simulink model "FSAC2021"  (R2014a)
settings: Solver=FixedStepDiscrete  StartTime=0.0  StopTime=inf  FixedStep=0.0005  RelTol=1e-3
model workspace (MAT data in the model file):
  MCOS : class17 (value not decoded)
  MCOS : class17 (value not decoded)
  MCOS : class17 (value not decoded)
  MCOS : class17 (value not decoded)
  MCOS : class17 (value not decoded)
  MCOS : class17 (value not decoded)
  MCOS : class17 (value not decoded)
  MCOS : class17 (value not decoded)
  MCOS : class17 (value not decoded)
  MCOS : class17 (value not decoded)
  MCOS : class17 (value not decoded)
  MCOS : class17 (value not decoded)
  MCOS : class17 (value not decoded)
  MCOS : class17 (value not decoded)
  MCOS : class17 (value not decoded)
  MCOS : class17 (value not decoded)
  MCOS : class17 (value not decoded)
  MCOS : class17 (value not decoded)
  MCOS : class17 (value not decoded)
  BUZZER_START = 1
  MCOS : class17 (value not decoded)
  MCOS : class17 (value not decoded)
  MCOS : class17 (value not decoded)
  MCOS : class17 (value not decoded)
  MCOS : class17 (value not decoded)
  MCOS : class17 (value not decoded)
  MCOS : class17 (value not decoded)
  MCOS : class17 (value not decoded)
  MCOS : class17 (value not decoded)
  MCOS : class17 (value not decoded)
  MCOS : class17 (value not decoded)
  MCOS : class17 (value not decoded)
  MCOS : class17 (value not decoded)
  MCOS : class17 (value not decoded)
  MCOS : class17 (value not decoded)
  MCOS : class17 (value not decoded)
  MCOS : class17 (value not decoded)
  MCOS : class17 (value not decoded)
  MCOS : class17 (value not decoded)
  MCOS : class17 (value not decoded)
  MCOS : class17 (value not decoded)
  MCOS : class17 (value not decoded)
  MCOS : class17 (value not decoded)
  MCOS : class17 (value not decoded)
  MCOS : class17 (value not decoded)
  MCOS : class17 (value not decoded)
  MCOS : class17 (value not decoded)
  MCOS : class17 (value not decoded)
  MCOS : class17 (value not decoded)
  MCOS : class17 (value not decoded)
  MCOS : class17 (value not decoded)
  MCOS : class17 (value not decoded)
  MCOS : class17 (value not decoded)
  MCOS : class17 (value not decoded)
  MCOS : class17 (value not decoded)
  MCOS : class17 (value not decoded)
  MCOS : class17 (value not decoded)
  MCOS : class17 (value not decoded)
  Brake = 11
  MCOS : class17 (value not decoded)
  MCOS : class17 (value not decoded)
  MCOS : class17 (value not decoded)
  MCOS : class17 (value not decoded)
  MCOS : class17 (value not decoded)
  MCOS : class17 (value not decoded)
  MCOS : class17 (value not decoded)
  MCOS : class17 (value not decoded)
  Sensor_Acc_b = 101.85
  Sensor_Acc_k = -0.0185
  Str_Sen_Orig_Angle = -341
  MCOS : class17 (value not decoded)
  Tire_D = 0.47
  T = 0.05
libraries: simulink x396, ec55xxlib x126
(part 16 of 17)

== system FSAC2021/ROUTING/TO_DCAN/Subsystem/DIAG_VEH_INFO/EBS_Gas_SN_1_Sts ==
  EBS_Gas_SN_1_Sts : Inport
  Constant{1..3,5..8} (7 alike) : Constant  Value=0  OutDataTypeStr=uint8  SampleTime=-1
  EBS_Gas_SN_1_StsRon : Rounding  Operator=round
  EBS_Gas_SN_1_Sts_1sat : Saturate  UpperLimit=16  LowerLimit=0
  EBS_Gas_SN_1_Sts_Convert : DataTypeConversion  OutDataTypeStr=uint8
  EBS_Gas_SN_1_Sts_Convert1 : DataTypeConversion  OutDataTypeStr=uint32
  EBS_Gas_SN_1_Sts_D : Product  Inputs=*/
  EBS_Gas_SN_1_Sts_F : Constant  OutDataTypeStr=single
  EBS_Gas_SN_1_Sts_L : simulink/Logic and Bit Operations/Bitwise Operator  logicop=AND  UseBitMask=on  BitMask=16  BitMaskRealWorld=Stored Integer
  EBS_Gas_SN_1_Sts_O : Constant  Value=0  OutDataTypeStr=single
  EBS_Gas_SN_1_Sts_S : ArithShift  BitShiftNumber=-4
  EBS_Gas_SN_1_Sts_sat : Saturate  UpperLimit=1  LowerLimit=0
  EBS_Gas_SN_1_Sts_st : Sum  Inputs=+-
  output1 : Outport
  output2 : Outport  Port=2
  output3 : Outport  Port=3
  output4 : Outport  Port=4
  output5 : Outport  Port=5
  output6 : Outport  Port=6
  output7 : Outport  Port=7
  output8 : Outport  Port=8
  wires:
  EBS_Gas_SN_1_Sts/1 -> EBS_Gas_SN_1_Sts_sat/1
  EBS_Gas_SN_1_Sts_sat/1 -> EBS_Gas_SN_1_Sts_st/1
  EBS_Gas_SN_1_Sts_O/1 -> EBS_Gas_SN_1_Sts_st/2
  EBS_Gas_SN_1_Sts_st/1 -> EBS_Gas_SN_1_Sts_D/1
  EBS_Gas_SN_1_Sts_F/1 -> EBS_Gas_SN_1_Sts_D/2
  EBS_Gas_SN_1_Sts_D/1 -> EBS_Gas_SN_1_StsRon/1
  EBS_Gas_SN_1_StsRon/1 -> EBS_Gas_SN_1_Sts_S/1
  EBS_Gas_SN_1_Sts_S/1 -> EBS_Gas_SN_1_Sts_1sat/1
  EBS_Gas_SN_1_Sts_1sat/1 -> EBS_Gas_SN_1_Sts_Convert1/1
  EBS_Gas_SN_1_Sts_Convert1/1 -> EBS_Gas_SN_1_Sts_L/1
  EBS_Gas_SN_1_Sts_L/1 -> EBS_Gas_SN_1_Sts_Convert/1
  EBS_Gas_SN_1_Sts_Convert/1 -> output4/1
  Constant1/1 -> output1/1
  Constant2/1 -> output2/1
  Constant3/1 -> output3/1
  Constant5/1 -> output5/1
  Constant6/1 -> output6/1
  Constant7/1 -> output7/1
  Constant8/1 -> output8/1

== system FSAC2021/ROUTING/TO_DCAN/Subsystem/DIAG_VEH_INFO/EBS_Gas_SN_2_Sts ==
  EBS_Gas_SN_2_Sts : Inport
  Constant{1..3,5..8} (7 alike) : Constant  Value=0  OutDataTypeStr=uint8  SampleTime=-1
  EBS_Gas_SN_2_StsRon : Rounding  Operator=round
  EBS_Gas_SN_2_Sts_1sat : Saturate  UpperLimit=8  LowerLimit=0
  EBS_Gas_SN_2_Sts_Convert : DataTypeConversion  OutDataTypeStr=uint8
  EBS_Gas_SN_2_Sts_Convert1 : DataTypeConversion  OutDataTypeStr=uint32
  EBS_Gas_SN_2_Sts_D : Product  Inputs=*/
  EBS_Gas_SN_2_Sts_F : Constant  OutDataTypeStr=single
  EBS_Gas_SN_2_Sts_L : simulink/Logic and Bit Operations/Bitwise Operator  logicop=AND  UseBitMask=on  BitMask=8  BitMaskRealWorld=Stored Integer
  EBS_Gas_SN_2_Sts_O : Constant  Value=0  OutDataTypeStr=single
  EBS_Gas_SN_2_Sts_S : ArithShift  BitShiftNumber=-3
  EBS_Gas_SN_2_Sts_sat : Saturate  UpperLimit=1  LowerLimit=0
  EBS_Gas_SN_2_Sts_st : Sum  Inputs=+-
  output1 : Outport
  output2 : Outport  Port=2
  output3 : Outport  Port=3
  output4 : Outport  Port=4
  output5 : Outport  Port=5
  output6 : Outport  Port=6
  output7 : Outport  Port=7
  output8 : Outport  Port=8
  wires:
  EBS_Gas_SN_2_Sts/1 -> EBS_Gas_SN_2_Sts_sat/1
  EBS_Gas_SN_2_Sts_sat/1 -> EBS_Gas_SN_2_Sts_st/1
  EBS_Gas_SN_2_Sts_O/1 -> EBS_Gas_SN_2_Sts_st/2
  EBS_Gas_SN_2_Sts_st/1 -> EBS_Gas_SN_2_Sts_D/1
  EBS_Gas_SN_2_Sts_F/1 -> EBS_Gas_SN_2_Sts_D/2
  EBS_Gas_SN_2_Sts_D/1 -> EBS_Gas_SN_2_StsRon/1
  EBS_Gas_SN_2_StsRon/1 -> EBS_Gas_SN_2_Sts_S/1
  EBS_Gas_SN_2_Sts_S/1 -> EBS_Gas_SN_2_Sts_1sat/1
  EBS_Gas_SN_2_Sts_1sat/1 -> EBS_Gas_SN_2_Sts_Convert1/1
  EBS_Gas_SN_2_Sts_Convert1/1 -> EBS_Gas_SN_2_Sts_L/1
  EBS_Gas_SN_2_Sts_L/1 -> EBS_Gas_SN_2_Sts_Convert/1
  EBS_Gas_SN_2_Sts_Convert/1 -> output4/1
  Constant1/1 -> output1/1
  Constant2/1 -> output2/1
  Constant3/1 -> output3/1
  Constant5/1 -> output5/1
  Constant6/1 -> output6/1
  Constant7/1 -> output7/1
  Constant8/1 -> output8/1

== system FSAC2021/ROUTING/TO_DCAN/Subsystem/DIAG_VEH_INFO/EBS_Rls_Switch ==
  EBS_Rls_Switch : Inport
  Constant{1,3..8} (7 alike) : Constant  Value=0  OutDataTypeStr=uint8  SampleTime=-1
  EBS_Rls_SwitchRon : Rounding  Operator=round
  EBS_Rls_Switch_1sat : Saturate  UpperLimit=8  LowerLimit=0
  EBS_Rls_Switch_Convert : DataTypeConversion  OutDataTypeStr=uint8
  EBS_Rls_Switch_Convert1 : DataTypeConversion  OutDataTypeStr=uint32
  EBS_Rls_Switch_D : Product  Inputs=*/
  EBS_Rls_Switch_F : Constant  OutDataTypeStr=single
  EBS_Rls_Switch_L : simulink/Logic and Bit Operations/Bitwise Operator  logicop=AND  UseBitMask=on  BitMask=8  BitMaskRealWorld=Stored Integer
  EBS_Rls_Switch_O : Constant  Value=0  OutDataTypeStr=single
  EBS_Rls_Switch_S : ArithShift  BitShiftNumber=-3
  EBS_Rls_Switch_sat : Saturate  UpperLimit=1  LowerLimit=0
  EBS_Rls_Switch_st : Sum  Inputs=+-
  output1 : Outport
  output2 : Outport  Port=2
  output3 : Outport  Port=3
  output4 : Outport  Port=4
  output5 : Outport  Port=5
  output6 : Outport  Port=6
  output7 : Outport  Port=7
  output8 : Outport  Port=8
  wires:
  EBS_Rls_Switch/1 -> EBS_Rls_Switch_sat/1
  EBS_Rls_Switch_sat/1 -> EBS_Rls_Switch_st/1
  EBS_Rls_Switch_O/1 -> EBS_Rls_Switch_st/2
  EBS_Rls_Switch_st/1 -> EBS_Rls_Switch_D/1
  EBS_Rls_Switch_F/1 -> EBS_Rls_Switch_D/2
  EBS_Rls_Switch_D/1 -> EBS_Rls_SwitchRon/1
  EBS_Rls_SwitchRon/1 -> EBS_Rls_Switch_S/1
  EBS_Rls_Switch_S/1 -> EBS_Rls_Switch_1sat/1
  EBS_Rls_Switch_1sat/1 -> EBS_Rls_Switch_Convert1/1
  EBS_Rls_Switch_Convert1/1 -> EBS_Rls_Switch_L/1
  EBS_Rls_Switch_L/1 -> EBS_Rls_Switch_Convert/1
  EBS_Rls_Switch_Convert/1 -> output2/1
  Constant1/1 -> output1/1
  Constant3/1 -> output3/1
  Constant4/1 -> output4/1
  Constant5/1 -> output5/1
  Constant6/1 -> output6/1
  Constant7/1 -> output7/1
  Constant8/1 -> output8/1

== system FSAC2021/ROUTING/TO_DCAN/Subsystem/DIAG_VEH_INFO/EBS_Status ==
  EBS_Status : Inport
  Constant{2..8} (7 alike) : Constant  Value=0  OutDataTypeStr=uint8  SampleTime=-1
  EBS_StatusRon : Rounding  Operator=round
  EBS_Status_1sat : Saturate  UpperLimit=192  LowerLimit=0
  EBS_Status_Convert : DataTypeConversion  OutDataTypeStr=uint8
  EBS_Status_Convert1 : DataTypeConversion  OutDataTypeStr=uint32
  EBS_Status_D : Product  Inputs=*/
  EBS_Status_F : Constant  OutDataTypeStr=single
  EBS_Status_L : simulink/Logic and Bit Operations/Bitwise Operator  logicop=AND  UseBitMask=on  BitMask=192  BitMaskRealWorld=Stored Integer
  EBS_Status_O : Constant  Value=0  OutDataTypeStr=single
  EBS_Status_S : ArithShift  BitShiftNumber=-6
  EBS_Status_sat : Saturate  UpperLimit=3  LowerLimit=0
  EBS_Status_st : Sum  Inputs=+-
  output1 : Outport
  output2 : Outport  Port=2
  output3 : Outport  Port=3
  output4 : Outport  Port=4
  output5 : Outport  Port=5
  output6 : Outport  Port=6
  output7 : Outport  Port=7
  output8 : Outport  Port=8
  wires:
  EBS_Status/1 -> EBS_Status_sat/1
  EBS_Status_sat/1 -> EBS_Status_st/1
  EBS_Status_O/1 -> EBS_Status_st/2
  EBS_Status_st/1 -> EBS_Status_D/1
  EBS_Status_F/1 -> EBS_Status_D/2
  EBS_Status_D/1 -> EBS_StatusRon/1
  EBS_StatusRon/1 -> EBS_Status_S/1
  EBS_Status_S/1 -> EBS_Status_1sat/1
  EBS_Status_1sat/1 -> EBS_Status_Convert1/1
  EBS_Status_Convert1/1 -> EBS_Status_L/1
  EBS_Status_L/1 -> EBS_Status_Convert/1
  EBS_Status_Convert/1 -> output1/1
  Constant2/1 -> output2/1
  Constant3/1 -> output3/1
  Constant4/1 -> output4/1
  Constant5/1 -> output5/1
  Constant6/1 -> output6/1
  Constant7/1 -> output7/1
  Constant8/1 -> output8/1

== system FSAC2021/ROUTING/TO_DCAN/Subsystem/DIAG_VEH_INFO/HV_Switch ==
  HV_Switch : Inport
  Constant{1,3..8} (7 alike) : Constant  Value=0  OutDataTypeStr=uint8  SampleTime=-1
  HV_SwitchRon : Rounding  Operator=round
  HV_Switch_1sat : Saturate  UpperLimit=16  LowerLimit=0
  HV_Switch_Convert : DataTypeConversion  OutDataTypeStr=uint8
  HV_Switch_Convert1 : DataTypeConversion  OutDataTypeStr=uint32
  HV_Switch_D : Product  Inputs=*/
  HV_Switch_F : Constant  OutDataTypeStr=single
  HV_Switch_L : simulink/Logic and Bit Operations/Bitwise Operator  logicop=AND  UseBitMask=on  BitMask=16  BitMaskRealWorld=Stored Integer
  HV_Switch_O : Constant  Value=0  OutDataTypeStr=single
  HV_Switch_S : ArithShift  BitShiftNumber=-4
  HV_Switch_sat : Saturate  UpperLimit=1  LowerLimit=0
  HV_Switch_st : Sum  Inputs=+-
  output1 : Outport
  output2 : Outport  Port=2
  output3 : Outport  Port=3
  output4 : Outport  Port=4
  output5 : Outport  Port=5
  output6 : Outport  Port=6
  output7 : Outport  Port=7
  output8 : Outport  Port=8
  wires:
  HV_Switch/1 -> HV_Switch_sat/1
  HV_Switch_sat/1 -> HV_Switch_st/1
  HV_Switch_O/1 -> HV_Switch_st/2
  HV_Switch_st/1 -> HV_Switch_D/1
  HV_Switch_F/1 -> HV_Switch_D/2
  HV_Switch_D/1 -> HV_SwitchRon/1
  HV_SwitchRon/1 -> HV_Switch_S/1
  HV_Switch_S/1 -> HV_Switch_1sat/1
  HV_Switch_1sat/1 -> HV_Switch_Convert1/1
  HV_Switch_Convert1/1 -> HV_Switch_L/1
  HV_Switch_L/1 -> HV_Switch_Convert/1
  HV_Switch_Convert/1 -> output2/1
  Constant1/1 -> output1/1
  Constant3/1 -> output3/1
  Constant4/1 -> output4/1
  Constant5/1 -> output5/1
  Constant6/1 -> output6/1
  Constant7/1 -> output7/1
  Constant8/1 -> output8/1

== system FSAC2021/ROUTING/TO_DCAN/Subsystem/DIAG_VEH_INFO/High_voltage_on ==
  High_voltage_on : Inport
  Constant{1,3..8} (7 alike) : Constant  Value=0  OutDataTypeStr=uint8  SampleTime=-1
  High_voltage_onRon : Rounding  Operator=round
  High_voltage_on_1sat : Saturate  UpperLimit=2  LowerLimit=0
  High_voltage_on_Convert : DataTypeConversion  OutDataTypeStr=uint8
  High_voltage_on_Convert1 : DataTypeConversion  OutDataTypeStr=uint32
  High_voltage_on_D : Product  Inputs=*/
  High_voltage_on_F : Constant  OutDataTypeStr=single
  High_voltage_on_L : simulink/Logic and Bit Operations/Bitwise Operator  logicop=AND  UseBitMask=on  BitMask=2  BitMaskRealWorld=Stored Integer
  High_voltage_on_O : Constant  Value=0  OutDataTypeStr=single
  High_voltage_on_S : ArithShift  BitShiftNumber=-1
  High_voltage_on_sat : Saturate  UpperLimit=1  LowerLimit=0
  High_voltage_on_st : Sum  Inputs=+-
  output1 : Outport
  output2 : Outport  Port=2
  output3 : Outport  Port=3
  output4 : Outport  Port=4
  output5 : Outport  Port=5
  output6 : Outport  Port=6
  output7 : Outport  Port=7
  output8 : Outport  Port=8
  wires:
  High_voltage_on/1 -> High_voltage_on_sat/1
  High_voltage_on_sat/1 -> High_voltage_on_st/1
  High_voltage_on_O/1 -> High_voltage_on_st/2
  High_voltage_on_st/1 -> High_voltage_on_D/1
  High_voltage_on_F/1 -> High_voltage_on_D/2
  High_voltage_on_D/1 -> High_voltage_onRon/1
  High_voltage_onRon/1 -> High_voltage_on_S/1
  High_voltage_on_S/1 -> High_voltage_on_1sat/1
  High_voltage_on_1sat/1 -> High_voltage_on_Convert1/1
  High_voltage_on_Convert1/1 -> High_voltage_on_L/1
  High_voltage_on_L/1 -> High_voltage_on_Convert/1
  High_voltage_on_Convert/1 -> output2/1
  Constant1/1 -> output1/1
  Constant3/1 -> output3/1
  Constant4/1 -> output4/1
  Constant5/1 -> output5/1
  Constant6/1 -> output6/1
  Constant7/1 -> output7/1
  Constant8/1 -> output8/1

== system FSAC2021/ROUTING/TO_DCAN/Subsystem/DIAG_VEH_INFO/Hydra_Prs_SN_Sts ==
  Hydra_Prs_SN_Sts : Inport
  Constant{2..8} (7 alike) : Constant  Value=0  OutDataTypeStr=uint8  SampleTime=-1
  Hydra_Prs_SN_StsRon : Rounding  Operator=round
  Hydra_Prs_SN_Sts_1sat : Saturate  UpperLimit=1  LowerLimit=0
  Hydra_Prs_SN_Sts_Convert : DataTypeConversion  OutDataTypeStr=uint8
  Hydra_Prs_SN_Sts_Convert1 : DataTypeConversion  OutDataTypeStr=uint32
  Hydra_Prs_SN_Sts_D : Product  Inputs=*/
  Hydra_Prs_SN_Sts_F : Constant  OutDataTypeStr=single
  Hydra_Prs_SN_Sts_L : simulink/Logic and Bit Operations/Bitwise Operator  logicop=AND  UseBitMask=on  BitMask=1  BitMaskRealWorld=Stored Integer
  Hydra_Prs_SN_Sts_O : Constant  Value=0  OutDataTypeStr=single
  Hydra_Prs_SN_Sts_S : ArithShift
  Hydra_Prs_SN_Sts_sat : Saturate  UpperLimit=1  LowerLimit=0
  Hydra_Prs_SN_Sts_st : Sum  Inputs=+-
  output1 : Outport
  output2 : Outport  Port=2
  output3 : Outport  Port=3
  output4 : Outport  Port=4
  output5 : Outport  Port=5
  output6 : Outport  Port=6
  output7 : Outport  Port=7
  output8 : Outport  Port=8
  wires:
  Hydra_Prs_SN_Sts/1 -> Hydra_Prs_SN_Sts_sat/1
  Hydra_Prs_SN_Sts_sat/1 -> Hydra_Prs_SN_Sts_st/1
  Hydra_Prs_SN_Sts_O/1 -> Hydra_Prs_SN_Sts_st/2
  Hydra_Prs_SN_Sts_st/1 -> Hydra_Prs_SN_Sts_D/1
  Hydra_Prs_SN_Sts_F/1 -> Hydra_Prs_SN_Sts_D/2
  Hydra_Prs_SN_Sts_D/1 -> Hydra_Prs_SN_StsRon/1
  Hydra_Prs_SN_StsRon/1 -> Hydra_Prs_SN_Sts_S/1
  Hydra_Prs_SN_Sts_S/1 -> Hydra_Prs_SN_Sts_1sat/1
  Hydra_Prs_SN_Sts_1sat/1 -> Hydra_Prs_SN_Sts_Convert1/1
  Hydra_Prs_SN_Sts_Convert1/1 -> Hydra_Prs_SN_Sts_L/1
  Hydra_Prs_SN_Sts_L/1 -> Hydra_Prs_SN_Sts_Convert/1
  Hydra_Prs_SN_Sts_Convert/1 -> output1/1
  Constant2/1 -> output2/1
  Constant3/1 -> output3/1
  Constant4/1 -> output4/1
  Constant5/1 -> output5/1
  Constant6/1 -> output6/1
  Constant7/1 -> output7/1
  Constant8/1 -> output8/1

== system FSAC2021/ROUTING/TO_DCAN/Subsystem/DIAG_VEH_INFO/LV_Switch ==
  LV_Switch : Inport
  Constant{1,3..8} (7 alike) : Constant  Value=0  OutDataTypeStr=uint8  SampleTime=-1
  LV_SwitchRon : Rounding  Operator=round
  LV_Switch_1sat : Saturate  UpperLimit=32  LowerLimit=0
  LV_Switch_Convert : DataTypeConversion  OutDataTypeStr=uint8
  LV_Switch_Convert1 : DataTypeConversion  OutDataTypeStr=uint32
  LV_Switch_D : Product  Inputs=*/
  LV_Switch_F : Constant  OutDataTypeStr=single
  LV_Switch_L : simulink/Logic and Bit Operations/Bitwise Operator  logicop=AND  UseBitMask=on  BitMask=32  BitMaskRealWorld=Stored Integer
  LV_Switch_O : Constant  Value=0  OutDataTypeStr=single
  LV_Switch_S : ArithShift  BitShiftNumber=-5
  LV_Switch_sat : Saturate  UpperLimit=1  LowerLimit=0
  LV_Switch_st : Sum  Inputs=+-
  output1 : Outport
  output2 : Outport  Port=2
  output3 : Outport  Port=3
  output4 : Outport  Port=4
  output5 : Outport  Port=5
  output6 : Outport  Port=6
  output7 : Outport  Port=7
  output8 : Outport  Port=8
  wires:
  LV_Switch/1 -> LV_Switch_sat/1
  LV_Switch_sat/1 -> LV_Switch_st/1
  LV_Switch_O/1 -> LV_Switch_st/2
  LV_Switch_st/1 -> LV_Switch_D/1
  LV_Switch_F/1 -> LV_Switch_D/2
  LV_Switch_D/1 -> LV_SwitchRon/1
  LV_SwitchRon/1 -> LV_Switch_S/1
  LV_Switch_S/1 -> LV_Switch_1sat/1
  LV_Switch_1sat/1 -> LV_Switch_Convert1/1
  LV_Switch_Convert1/1 -> LV_Switch_L/1
  LV_Switch_L/1 -> LV_Switch_Convert/1
  LV_Switch_Convert/1 -> output2/1
  Constant1/1 -> output1/1
  Constant3/1 -> output3/1
  Constant4/1 -> output4/1
  Constant5/1 -> output5/1
  Constant6/1 -> output6/1
  Constant7/1 -> output7/1
  Constant8/1 -> output8/1

== system FSAC2021/ROUTING/TO_DCAN/Subsystem/DIAG_VEH_INFO/On_In_Swtich ==
  On_In_Swtich : Inport
  Constant{1,3..8} (7 alike) : Constant  Value=0  OutDataTypeStr=uint8  SampleTime=-1
  On_In_SwtichRon : Rounding  Operator=round
  On_In_Swtich_1sat : Saturate  UpperLimit=64  LowerLimit=0
  On_In_Swtich_Convert : DataTypeConversion  OutDataTypeStr=uint8
  On_In_Swtich_Convert1 : DataTypeConversion  OutDataTypeStr=uint32
  On_In_Swtich_D : Product  Inputs=*/
  On_In_Swtich_F : Constant  OutDataTypeStr=single
  On_In_Swtich_L : simulink/Logic and Bit Operations/Bitwise Operator  logicop=AND  UseBitMask=on  BitMask=64  BitMaskRealWorld=Stored Integer
  On_In_Swtich_O : Constant  Value=0  OutDataTypeStr=single
  On_In_Swtich_S : ArithShift  BitShiftNumber=-6
  On_In_Swtich_sat : Saturate  UpperLimit=1  LowerLimit=0
  On_In_Swtich_st : Sum  Inputs=+-
  output1 : Outport
  output2 : Outport  Port=2
  output3 : Outport  Port=3
  output4 : Outport  Port=4
  output5 : Outport  Port=5
  output6 : Outport  Port=6
  output7 : Outport  Port=7
  output8 : Outport  Port=8
  wires:
  On_In_Swtich/1 -> On_In_Swtich_sat/1
  On_In_Swtich_sat/1 -> On_In_Swtich_st/1
  On_In_Swtich_O/1 -> On_In_Swtich_st/2
  On_In_Swtich_st/1 -> On_In_Swtich_D/1
  On_In_Swtich_F/1 -> On_In_Swtich_D/2
  On_In_Swtich_D/1 -> On_In_SwtichRon/1
  On_In_SwtichRon/1 -> On_In_Swtich_S/1
  On_In_Swtich_S/1 -> On_In_Swtich_1sat/1
  On_In_Swtich_1sat/1 -> On_In_Swtich_Convert1/1
  On_In_Swtich_Convert1/1 -> On_In_Swtich_L/1
  On_In_Swtich_L/1 -> On_In_Swtich_Convert/1
  On_In_Swtich_Convert/1 -> output2/1
  Constant1/1 -> output1/1
  Constant3/1 -> output3/1
  Constant4/1 -> output4/1
  Constant5/1 -> output5/1
  Constant6/1 -> output6/1
  Constant7/1 -> output7/1
  Constant8/1 -> output8/1

== system FSAC2021/ROUTING/TO_DCAN/Subsystem/DIAG_VEH_INFO/On_Out_Switch ==
  On_Out_Switch : Inport
  Constant{1,3..8} (7 alike) : Constant  Value=0  OutDataTypeStr=uint8  SampleTime=-1
  On_Out_SwitchRon : Rounding  Operator=round
  On_Out_Switch_1sat : Saturate  UpperLimit=128  LowerLimit=0
  On_Out_Switch_Convert : DataTypeConversion  OutDataTypeStr=uint8
  On_Out_Switch_Convert1 : DataTypeConversion  OutDataTypeStr=uint32
  On_Out_Switch_D : Product  Inputs=*/
  On_Out_Switch_F : Constant  OutDataTypeStr=single
  On_Out_Switch_L : simulink/Logic and Bit Operations/Bitwise Operator  logicop=AND  UseBitMask=on  BitMask=128  BitMaskRealWorld=Stored Integer
  On_Out_Switch_O : Constant  Value=0  OutDataTypeStr=single
  On_Out_Switch_S : ArithShift  BitShiftNumber=-7
  On_Out_Switch_sat : Saturate  UpperLimit=1  LowerLimit=0
  On_Out_Switch_st : Sum  Inputs=+-
  output1 : Outport
  output2 : Outport  Port=2
  output3 : Outport  Port=3
  output4 : Outport  Port=4
  output5 : Outport  Port=5
  output6 : Outport  Port=6
  output7 : Outport  Port=7
  output8 : Outport  Port=8
  wires:
  On_Out_Switch/1 -> On_Out_Switch_sat/1
  On_Out_Switch_sat/1 -> On_Out_Switch_st/1
  On_Out_Switch_O/1 -> On_Out_Switch_st/2
  On_Out_Switch_st/1 -> On_Out_Switch_D/1
  On_Out_Switch_F/1 -> On_Out_Switch_D/2
  On_Out_Switch_D/1 -> On_Out_SwitchRon/1
  On_Out_SwitchRon/1 -> On_Out_Switch_S/1
  On_Out_Switch_S/1 -> On_Out_Switch_1sat/1
  On_Out_Switch_1sat/1 -> On_Out_Switch_Convert1/1
  On_Out_Switch_Convert1/1 -> On_Out_Switch_L/1
  On_Out_Switch_L/1 -> On_Out_Switch_Convert/1
  On_Out_Switch_Convert/1 -> output2/1
  Constant1/1 -> output1/1
  Constant3/1 -> output3/1
  Constant4/1 -> output4/1
  Constant5/1 -> output5/1
  Constant6/1 -> output6/1
  Constant7/1 -> output7/1
  Constant8/1 -> output8/1

== system FSAC2021/ROUTING/TO_DCAN/Subsystem/DIAG_VEH_INFO/Point_BCU ==
  Point_BCU : Inport
  Constant{1..2,4..8} (7 alike) : Constant  Value=0  OutDataTypeStr=uint8  SampleTime=-1
  Point_BCURon : Rounding  Operator=round
  Point_BCU_1sat : Saturate  UpperLimit=32  LowerLimit=0
  Point_BCU_Convert : DataTypeConversion  OutDataTypeStr=uint8
  Point_BCU_Convert1 : DataTypeConversion  OutDataTypeStr=uint32
  Point_BCU_D : Product  Inputs=*/
  Point_BCU_F : Constant  OutDataTypeStr=single
  Point_BCU_L : simulink/Logic and Bit Operations/Bitwise Operator  logicop=AND  UseBitMask=on  BitMask=32  BitMaskRealWorld=Stored Integer
  Point_BCU_O : Constant  Value=0  OutDataTypeStr=single
  Point_BCU_S : ArithShift  BitShiftNumber=-5
  Point_BCU_sat : Saturate  UpperLimit=1  LowerLimit=0
  Point_BCU_st : Sum  Inputs=+-
  output1 : Outport
  output2 : Outport  Port=2
  output3 : Outport  Port=3
  output4 : Outport  Port=4
  output5 : Outport  Port=5
  output6 : Outport  Port=6
  output7 : Outport  Port=7
  output8 : Outport  Port=8
  wires:
  Point_BCU/1 -> Point_BCU_sat/1
  Point_BCU_sat/1 -> Point_BCU_st/1
  Point_BCU_O/1 -> Point_BCU_st/2
  Point_BCU_st/1 -> Point_BCU_D/1
  Point_BCU_F/1 -> Point_BCU_D/2
  Point_BCU_D/1 -> Point_BCURon/1
  Point_BCURon/1 -> Point_BCU_S/1
  Point_BCU_S/1 -> Point_BCU_1sat/1
  Point_BCU_1sat/1 -> Point_BCU_Convert1/1
  Point_BCU_Convert1/1 -> Point_BCU_L/1
  Point_BCU_L/1 -> Point_BCU_Convert/1
  Point_BCU_Convert/1 -> output3/1
  Constant1/1 -> output1/1
  Constant2/1 -> output2/1
  Constant4/1 -> output4/1
  Constant5/1 -> output5/1
  Constant6/1 -> output6/1
  Constant7/1 -> output7/1
  Constant8/1 -> output8/1

== system FSAC2021/ROUTING/TO_DCAN/Subsystem/DIAG_VEH_INFO/Point_BMS ==
  Point_BMS : Inport
  Constant{1..2,4..8} (7 alike) : Constant  Value=0  OutDataTypeStr=uint8  SampleTime=-1
  Point_BMSRon : Rounding  Operator=round
  Point_BMS_1sat : Saturate  UpperLimit=16  LowerLimit=0
  Point_BMS_Convert : DataTypeConversion  OutDataTypeStr=uint8
  Point_BMS_Convert1 : DataTypeConversion  OutDataTypeStr=uint32
  Point_BMS_D : Product  Inputs=*/
  Point_BMS_F : Constant  OutDataTypeStr=single
  Point_BMS_L : simulink/Logic and Bit Operations/Bitwise Operator  logicop=AND  UseBitMask=on  BitMask=16  BitMaskRealWorld=Stored Integer
  Point_BMS_O : Constant  Value=0  OutDataTypeStr=single
  Point_BMS_S : ArithShift  BitShiftNumber=-4
  Point_BMS_sat : Saturate  UpperLimit=1  LowerLimit=0
  Point_BMS_st : Sum  Inputs=+-
  output1 : Outport
  output2 : Outport  Port=2
  output3 : Outport  Port=3
  output4 : Outport  Port=4
  output5 : Outport  Port=5
  output6 : Outport  Port=6
  output7 : Outport  Port=7
  output8 : Outport  Port=8
  wires:
  Point_BMS/1 -> Point_BMS_sat/1
  Point_BMS_sat/1 -> Point_BMS_st/1
  Point_BMS_O/1 -> Point_BMS_st/2
  Point_BMS_st/1 -> Point_BMS_D/1
  Point_BMS_F/1 -> Point_BMS_D/2
  Point_BMS_D/1 -> Point_BMSRon/1
  Point_BMSRon/1 -> Point_BMS_S/1
  Point_BMS_S/1 -> Point_BMS_1sat/1
  Point_BMS_1sat/1 -> Point_BMS_Convert1/1
  Point_BMS_Convert1/1 -> Point_BMS_L/1
  Point_BMS_L/1 -> Point_BMS_Convert/1
  Point_BMS_Convert/1 -> output3/1
  Constant1/1 -> output1/1
  Constant2/1 -> output2/1
  Constant4/1 -> output4/1
  Constant5/1 -> output5/1
  Constant6/1 -> output6/1
  Constant7/1 -> output7/1
  Constant8/1 -> output8/1

== system FSAC2021/ROUTING/TO_DCAN/Subsystem/DIAG_VEH_INFO/Point_Drive_Motor ==
  Point_Drive_Motor : Inport
  Constant{1..2,4..8} (7 alike) : Constant  Value=0  OutDataTypeStr=uint8  SampleTime=-1
  Point_Drive_MotorRon : Rounding  Operator=round
  Point_Drive_Motor_1sat : Saturate  UpperLimit=8  LowerLimit=0
  Point_Drive_Motor_Convert : DataTypeConversion  OutDataTypeStr=uint8
  Point_Drive_Motor_Convert1 : DataTypeConversion  OutDataTypeStr=uint32
  Point_Drive_Motor_D : Product  Inputs=*/
  Point_Drive_Motor_F : Constant  OutDataTypeStr=single
  Point_Drive_Motor_L : simulink/Logic and Bit Operations/Bitwise Operator  logicop=AND  UseBitMask=on  BitMask=8  BitMaskRealWorld=Stored Integer
  Point_Drive_Motor_O : Constant  Value=0  OutDataTypeStr=single
  Point_Drive_Motor_S : ArithShift  BitShiftNumber=-3
  Point_Drive_Motor_sat : Saturate  UpperLimit=1  LowerLimit=0
  Point_Drive_Motor_st : Sum  Inputs=+-
  output1 : Outport
  output2 : Outport  Port=2
  output3 : Outport  Port=3
  output4 : Outport  Port=4
  output5 : Outport  Port=5
  output6 : Outport  Port=6
  output7 : Outport  Port=7
  output8 : Outport  Port=8
  wires:
  Point_Drive_Motor/1 -> Point_Drive_Motor_sat/1
  Point_Drive_Motor_sat/1 -> Point_Drive_Motor_st/1
  Point_Drive_Motor_O/1 -> Point_Drive_Motor_st/2
  Point_Drive_Motor_st/1 -> Point_Drive_Motor_D/1
  Point_Drive_Motor_F/1 -> Point_Drive_Motor_D/2
  Point_Drive_Motor_D/1 -> Point_Drive_MotorRon/1
  Point_Drive_MotorRon/1 -> Point_Drive_Motor_S/1
  Point_Drive_Motor_S/1 -> Point_Drive_Motor_1sat/1
  Point_Drive_Motor_1sat/1 -> Point_Drive_Motor_Convert1/1
  Point_Drive_Motor_Convert1/1 -> Point_Drive_Motor_L/1
  Point_Drive_Motor_L/1 -> Point_Drive_Motor_Convert/1
  Point_Drive_Motor_Convert/1 -> output3/1
  Constant1/1 -> output1/1
  Constant2/1 -> output2/1
  Constant4/1 -> output4/1
  Constant5/1 -> output5/1
  Constant6/1 -> output6/1
  Constant7/1 -> output7/1
  Constant8/1 -> output8/1

== system FSAC2021/ROUTING/TO_DCAN/Subsystem/DIAG_VEH_INFO/Point_IPC ==
  Point_IPC : Inport
  Constant{1..2,4..8} (7 alike) : Constant  Value=0  OutDataTypeStr=uint8  SampleTime=-1
  Point_IPCRon : Rounding  Operator=round
  Point_IPC_1sat : Saturate  UpperLimit=4  LowerLimit=0
  Point_IPC_Convert : DataTypeConversion  OutDataTypeStr=uint8
  Point_IPC_Convert1 : DataTypeConversion  OutDataTypeStr=uint32
  Point_IPC_D : Product  Inputs=*/
  Point_IPC_F : Constant  OutDataTypeStr=single
  Point_IPC_L : simulink/Logic and Bit Operations/Bitwise Operator  logicop=AND  UseBitMask=on  BitMask=4  BitMaskRealWorld=Stored Integer
  Point_IPC_O : Constant  Value=0  OutDataTypeStr=single
  Point_IPC_S : ArithShift  BitShiftNumber=-2
  Point_IPC_sat : Saturate  UpperLimit=1  LowerLimit=0
  Point_IPC_st : Sum  Inputs=+-
  output1 : Outport
  output2 : Outport  Port=2
  output3 : Outport  Port=3
  output4 : Outport  Port=4
  output5 : Outport  Port=5
  output6 : Outport  Port=6
  output7 : Outport  Port=7
  output8 : Outport  Port=8
  wires:
  Point_IPC/1 -> Point_IPC_sat/1
  Point_IPC_sat/1 -> Point_IPC_st/1
  Point_IPC_O/1 -> Point_IPC_st/2
  Point_IPC_st/1 -> Point_IPC_D/1
  Point_IPC_F/1 -> Point_IPC_D/2
  Point_IPC_D/1 -> Point_IPCRon/1
  Point_IPCRon/1 -> Point_IPC_S/1
  Point_IPC_S/1 -> Point_IPC_1sat/1
  Point_IPC_1sat/1 -> Point_IPC_Convert1/1
  Point_IPC_Convert1/1 -> Point_IPC_L/1
  Point_IPC_L/1 -> Point_IPC_Convert/1
  Point_IPC_Convert/1 -> output3/1
  Constant1/1 -> output1/1
  Constant2/1 -> output2/1
  Constant4/1 -> output4/1
  Constant5/1 -> output5/1
  Constant6/1 -> output6/1
  Constant7/1 -> output7/1
  Constant8/1 -> output8/1

== system FSAC2021/ROUTING/TO_DCAN/Subsystem/DIAG_VEH_INFO/Point_MCU ==
  Point_MCU : Inport
  Constant{1..2,4..8} (7 alike) : Constant  Value=0  OutDataTypeStr=uint8  SampleTime=-1
  Point_MCURon : Rounding  Operator=round
  Point_MCU_1sat : Saturate  UpperLimit=2  LowerLimit=0
  Point_MCU_Convert : DataTypeConversion  OutDataTypeStr=uint8
  Point_MCU_Convert1 : DataTypeConversion  OutDataTypeStr=uint32
  Point_MCU_D : Product  Inputs=*/
  Point_MCU_F : Constant  OutDataTypeStr=single
  Point_MCU_L : simulink/Logic and Bit Operations/Bitwise Operator  logicop=AND  UseBitMask=on  BitMask=2  BitMaskRealWorld=Stored Integer
  Point_MCU_O : Constant  Value=0  OutDataTypeStr=single
  Point_MCU_S : ArithShift  BitShiftNumber=-1
  Point_MCU_sat : Saturate  UpperLimit=1  LowerLimit=0
  Point_MCU_st : Sum  Inputs=+-
  output1 : Outport
  output2 : Outport  Port=2
  output3 : Outport  Port=3
  output4 : Outport  Port=4
  output5 : Outport  Port=5
  output6 : Outport  Port=6
  output7 : Outport  Port=7
  output8 : Outport  Port=8
  wires:
  Point_MCU/1 -> Point_MCU_sat/1
  Point_MCU_sat/1 -> Point_MCU_st/1
  Point_MCU_O/1 -> Point_MCU_st/2
  Point_MCU_st/1 -> Point_MCU_D/1
  Point_MCU_F/1 -> Point_MCU_D/2
  Point_MCU_D/1 -> Point_MCURon/1
  Point_MCURon/1 -> Point_MCU_S/1
  Point_MCU_S/1 -> Point_MCU_1sat/1
  Point_MCU_1sat/1 -> Point_MCU_Convert1/1
  Point_MCU_Convert1/1 -> Point_MCU_L/1
  Point_MCU_L/1 -> Point_MCU_Convert/1
  Point_MCU_Convert/1 -> output3/1
  Constant1/1 -> output1/1
  Constant2/1 -> output2/1
  Constant4/1 -> output4/1
  Constant5/1 -> output5/1
  Constant6/1 -> output6/1
  Constant7/1 -> output7/1
  Constant8/1 -> output8/1

== system FSAC2021/ROUTING/TO_DCAN/Subsystem/DIAG_VEH_INFO/Point_RES ==
  Point_RES : Inport
  Constant{1..2,4..8} (7 alike) : Constant  Value=0  OutDataTypeStr=uint8  SampleTime=-1
  Point_RESRon : Rounding  Operator=round
  Point_RES_1sat : Saturate  UpperLimit=1  LowerLimit=0
  Point_RES_Convert : DataTypeConversion  OutDataTypeStr=uint8
  Point_RES_Convert1 : DataTypeConversion  OutDataTypeStr=uint32
  Point_RES_D : Product  Inputs=*/
  Point_RES_F : Constant  OutDataTypeStr=single
  Point_RES_L : simulink/Logic and Bit Operations/Bitwise Operator  logicop=AND  UseBitMask=on  BitMask=1  BitMaskRealWorld=Stored Integer
  Point_RES_O : Constant  Value=0  OutDataTypeStr=single
  Point_RES_S : ArithShift
  Point_RES_sat : Saturate  UpperLimit=1  LowerLimit=0
  Point_RES_st : Sum  Inputs=+-
  output1 : Outport
  output2 : Outport  Port=2
  output3 : Outport  Port=3
  output4 : Outport  Port=4
  output5 : Outport  Port=5
  output6 : Outport  Port=6
  output7 : Outport  Port=7
  output8 : Outport  Port=8
  wires:
  Point_RES/1 -> Point_RES_sat/1
  Point_RES_sat/1 -> Point_RES_st/1
  Point_RES_O/1 -> Point_RES_st/2
  Point_RES_st/1 -> Point_RES_D/1
  Point_RES_F/1 -> Point_RES_D/2
  Point_RES_D/1 -> Point_RESRon/1
  Point_RESRon/1 -> Point_RES_S/1
  Point_RES_S/1 -> Point_RES_1sat/1
  Point_RES_1sat/1 -> Point_RES_Convert1/1
  Point_RES_Convert1/1 -> Point_RES_L/1
  Point_RES_L/1 -> Point_RES_Convert/1
  Point_RES_Convert/1 -> output3/1
  Constant1/1 -> output1/1
  Constant2/1 -> output2/1
  Constant4/1 -> output4/1
  Constant5/1 -> output5/1
  Constant6/1 -> output6/1
  Constant7/1 -> output7/1
  Constant8/1 -> output8/1

== system FSAC2021/ROUTING/TO_DCAN/Subsystem/DIAG_VEH_INFO/Point_SCU ==
  Point_SCU : Inport
  Constant{1..3,5..8} (7 alike) : Constant  Value=0  OutDataTypeStr=uint8  SampleTime=-1
  Point_SCURon : Rounding  Operator=round
  Point_SCU_1sat : Saturate  UpperLimit=2  LowerLimit=0
  Point_SCU_Convert : DataTypeConversion  OutDataTypeStr=uint8
  Point_SCU_Convert1 : DataTypeConversion  OutDataTypeStr=uint32
  Point_SCU_D : Product  Inputs=*/
  Point_SCU_F : Constant  OutDataTypeStr=single
  Point_SCU_L : simulink/Logic and Bit Operations/Bitwise Operator  logicop=AND  UseBitMask=on  BitMask=2  BitMaskRealWorld=Stored Integer
  Point_SCU_O : Constant  Value=0  OutDataTypeStr=single
  Point_SCU_S : ArithShift  BitShiftNumber=-1
  Point_SCU_sat : Saturate  UpperLimit=1  LowerLimit=0
  Point_SCU_st : Sum  Inputs=+-
  output1 : Outport
  output2 : Outport  Port=2
  output3 : Outport  Port=3
  output4 : Outport  Port=4
  output5 : Outport  Port=5
  output6 : Outport  Port=6
  output7 : Outport  Port=7
  output8 : Outport  Port=8
  wires:
  Point_SCU/1 -> Point_SCU_sat/1
  Point_SCU_sat/1 -> Point_SCU_st/1
  Point_SCU_O/1 -> Point_SCU_st/2
  Point_SCU_st/1 -> Point_SCU_D/1
  Point_SCU_F/1 -> Point_SCU_D/2
  Point_SCU_D/1 -> Point_SCURon/1
  Point_SCURon/1 -> Point_SCU_S/1
  Point_SCU_S/1 -> Point_SCU_1sat/1
  Point_SCU_1sat/1 -> Point_SCU_Convert1/1
  Point_SCU_Convert1/1 -> Point_SCU_L/1
  Point_SCU_L/1 -> Point_SCU_Convert/1
  Point_SCU_Convert/1 -> output4/1
  Constant1/1 -> output1/1
  Constant2/1 -> output2/1
  Constant3/1 -> output3/1
  Constant5/1 -> output5/1
  Constant6/1 -> output6/1
  Constant7/1 -> output7/1
  Constant8/1 -> output8/1

== system FSAC2021/ROUTING/TO_DCAN/Subsystem/DIAG_VEH_INFO/Point_StrSr ==
  Point_StrSr : Inport
  Constant{1..3,5..8} (7 alike) : Constant  Value=0  OutDataTypeStr=uint8  SampleTime=-1
  Point_StrSrRon : Rounding  Operator=round
  Point_StrSr_1sat : Saturate  UpperLimit=1  LowerLimit=0
  Point_StrSr_Convert : DataTypeConversion  OutDataTypeStr=uint8
  Point_StrSr_Convert1 : DataTypeConversion  OutDataTypeStr=uint32
  Point_StrSr_D : Product  Inputs=*/
  Point_StrSr_F : Constant  OutDataTypeStr=single
  Point_StrSr_L : simulink/Logic and Bit Operations/Bitwise Operator  logicop=AND  UseBitMask=on  BitMask=1  BitMaskRealWorld=Stored Integer
  Point_StrSr_O : Constant  Value=0  OutDataTypeStr=single
  Point_StrSr_S : ArithShift
  Point_StrSr_sat : Saturate  UpperLimit=1  LowerLimit=0
  Point_StrSr_st : Sum  Inputs=+-
  output1 : Outport
  output2 : Outport  Port=2
  output3 : Outport  Port=3
  output4 : Outport  Port=4
  output5 : Outport  Port=5
  output6 : Outport  Port=6
  output7 : Outport  Port=7
  output8 : Outport  Port=8
  wires:
  Point_StrSr/1 -> Point_StrSr_sat/1
  Point_StrSr_sat/1 -> Point_StrSr_st/1
  Point_StrSr_O/1 -> Point_StrSr_st/2
  Point_StrSr_st/1 -> Point_StrSr_D/1
  Point_StrSr_F/1 -> Point_StrSr_D/2
  Point_StrSr_D/1 -> Point_StrSrRon/1
  Point_StrSrRon/1 -> Point_StrSr_S/1
  Point_StrSr_S/1 -> Point_StrSr_1sat/1
  Point_StrSr_1sat/1 -> Point_StrSr_Convert1/1
  Point_StrSr_Convert1/1 -> Point_StrSr_L/1
  Point_StrSr_L/1 -> Point_StrSr_Convert/1
  Point_StrSr_Convert/1 -> output4/1
  Constant1/1 -> output1/1
  Constant2/1 -> output2/1
  Constant3/1 -> output3/1
  Constant5/1 -> output5/1
  Constant6/1 -> output6/1
  Constant7/1 -> output7/1
  Constant8/1 -> output8/1

== system FSAC2021/ROUTING/TO_DCAN/Subsystem/DIAG_VEH_INFO/Point_VCU ==
  Point_VCU : Inport
  Constant{1..2,4..8} (7 alike) : Constant  Value=0  OutDataTypeStr=uint8  SampleTime=-1
  Point_VCURon : Rounding  Operator=round
  Point_VCU_1sat : Saturate  UpperLimit=128  LowerLimit=0
  Point_VCU_Convert : DataTypeConversion  OutDataTypeStr=uint8
  Point_VCU_Convert1 : DataTypeConversion  OutDataTypeStr=uint32
  Point_VCU_D : Product  Inputs=*/
  Point_VCU_F : Constant  OutDataTypeStr=single
  Point_VCU_L : simulink/Logic and Bit Operations/Bitwise Operator  logicop=AND  UseBitMask=on  BitMask=128  BitMaskRealWorld=Stored Integer
  Point_VCU_O : Constant  Value=0  OutDataTypeStr=single
  Point_VCU_S : ArithShift  BitShiftNumber=-7
  Point_VCU_sat : Saturate  UpperLimit=1  LowerLimit=0
  Point_VCU_st : Sum  Inputs=+-
  output1 : Outport
  output2 : Outport  Port=2
  output3 : Outport  Port=3
  output4 : Outport  Port=4
  output5 : Outport  Port=5
  output6 : Outport  Port=6
  output7 : Outport  Port=7
  output8 : Outport  Port=8
  wires:
  Point_VCU/1 -> Point_VCU_sat/1
  Point_VCU_sat/1 -> Point_VCU_st/1
  Point_VCU_O/1 -> Point_VCU_st/2
  Point_VCU_st/1 -> Point_VCU_D/1
  Point_VCU_F/1 -> Point_VCU_D/2
  Point_VCU_D/1 -> Point_VCURon/1
  Point_VCURon/1 -> Point_VCU_S/1
  Point_VCU_S/1 -> Point_VCU_1sat/1
  Point_VCU_1sat/1 -> Point_VCU_Convert1/1
  Point_VCU_Convert1/1 -> Point_VCU_L/1
  Point_VCU_L/1 -> Point_VCU_Convert/1
  Point_VCU_Convert/1 -> output3/1
  Constant1/1 -> output1/1
  Constant2/1 -> output2/1
  Constant4/1 -> output4/1
  Constant5/1 -> output5/1
  Constant6/1 -> output6/1
  Constant7/1 -> output7/1
  Constant8/1 -> output8/1

== system FSAC2021/ROUTING/TO_DCAN/Subsystem/DIAG_VEH_INFO/Start_Swtich ==
  Start_Swtich : Inport
  Constant{1..2,4..8} (7 alike) : Constant  Value=0  OutDataTypeStr=uint8  SampleTime=-1
  Start_SwtichRon : Rounding  Operator=round
  Start_Swtich_1sat : Saturate  UpperLimit=64  LowerLimit=0
  Start_Swtich_Convert : DataTypeConversion  OutDataTypeStr=uint8
  Start_Swtich_Convert1 : DataTypeConversion  OutDataTypeStr=uint32
  Start_Swtich_D : Product  Inputs=*/
  Start_Swtich_F : Constant  OutDataTypeStr=single
  Start_Swtich_L : simulink/Logic and Bit Operations/Bitwise Operator  logicop=AND  UseBitMask=on  BitMask=64  BitMaskRealWorld=Stored Integer
  Start_Swtich_O : Constant  Value=0  OutDataTypeStr=single
  Start_Swtich_S : ArithShift  BitShiftNumber=-6
  Start_Swtich_sat : Saturate  UpperLimit=1  LowerLimit=0
  Start_Swtich_st : Sum  Inputs=+-
  output1 : Outport
  output2 : Outport  Port=2
  output3 : Outport  Port=3
  output4 : Outport  Port=4
  output5 : Outport  Port=5
  output6 : Outport  Port=6
  output7 : Outport  Port=7
  output8 : Outport  Port=8
  wires:
  Start_Swtich/1 -> Start_Swtich_sat/1
  Start_Swtich_sat/1 -> Start_Swtich_st/1
  Start_Swtich_O/1 -> Start_Swtich_st/2
  Start_Swtich_st/1 -> Start_Swtich_D/1
  Start_Swtich_F/1 -> Start_Swtich_D/2
  Start_Swtich_D/1 -> Start_SwtichRon/1
  Start_SwtichRon/1 -> Start_Swtich_S/1
  Start_Swtich_S/1 -> Start_Swtich_1sat/1
  Start_Swtich_1sat/1 -> Start_Swtich_Convert1/1
  Start_Swtich_Convert1/1 -> Start_Swtich_L/1
  Start_Swtich_L/1 -> Start_Swtich_Convert/1
  Start_Swtich_Convert/1 -> output3/1
  Constant1/1 -> output1/1
  Constant2/1 -> output2/1
  Constant4/1 -> output4/1
  Constant5/1 -> output5/1
  Constant6/1 -> output6/1
  Constant7/1 -> output7/1
  Constant8/1 -> output8/1

== system FSAC2021/ROUTING/TO_DCAN/Subsystem/DIAG_VEH_INFO/Volt_Cmp_BMS_Sts ==
  Volt_Cmp_BMS_Sts : Inport
  Constant{1..3,5..8} (7 alike) : Constant  Value=0  OutDataTypeStr=uint8  SampleTime=-1
  Volt_Cmp_BMS_StsRon : Rounding  Operator=round
  Volt_Cmp_BMS_Sts_1sat : Saturate  UpperLimit=4  LowerLimit=0
  Volt_Cmp_BMS_Sts_Convert : DataTypeConversion  OutDataTypeStr=uint8
  Volt_Cmp_BMS_Sts_Convert1 : DataTypeConversion  OutDataTypeStr=uint32
  Volt_Cmp_BMS_Sts_D : Product  Inputs=*/
  Volt_Cmp_BMS_Sts_F : Constant  OutDataTypeStr=single
  Volt_Cmp_BMS_Sts_L : simulink/Logic and Bit Operations/Bitwise Operator  logicop=AND  UseBitMask=on  BitMask=4  BitMaskRealWorld=Stored Integer
  Volt_Cmp_BMS_Sts_O : Constant  Value=0  OutDataTypeStr=single
  Volt_Cmp_BMS_Sts_S : ArithShift  BitShiftNumber=-2
  Volt_Cmp_BMS_Sts_sat : Saturate  UpperLimit=1  LowerLimit=0
  Volt_Cmp_BMS_Sts_st : Sum  Inputs=+-
  output1 : Outport
  output2 : Outport  Port=2
  output3 : Outport  Port=3
  output4 : Outport  Port=4
  output5 : Outport  Port=5
  output6 : Outport  Port=6
  output7 : Outport  Port=7
  output8 : Outport  Port=8
  wires:
  Volt_Cmp_BMS_Sts/1 -> Volt_Cmp_BMS_Sts_sat/1
  Volt_Cmp_BMS_Sts_sat/1 -> Volt_Cmp_BMS_Sts_st/1
  Volt_Cmp_BMS_Sts_O/1 -> Volt_Cmp_BMS_Sts_st/2
  Volt_Cmp_BMS_Sts_st/1 -> Volt_Cmp_BMS_Sts_D/1
  Volt_Cmp_BMS_Sts_F/1 -> Volt_Cmp_BMS_Sts_D/2
  Volt_Cmp_BMS_Sts_D/1 -> Volt_Cmp_BMS_StsRon/1
  Volt_Cmp_BMS_StsRon/1 -> Volt_Cmp_BMS_Sts_S/1
  Volt_Cmp_BMS_Sts_S/1 -> Volt_Cmp_BMS_Sts_1sat/1
  Volt_Cmp_BMS_Sts_1sat/1 -> Volt_Cmp_BMS_Sts_Convert1/1
  Volt_Cmp_BMS_Sts_Convert1/1 -> Volt_Cmp_BMS_Sts_L/1
  Volt_Cmp_BMS_Sts_L/1 -> Volt_Cmp_BMS_Sts_Convert/1
  Volt_Cmp_BMS_Sts_Convert/1 -> output4/1
  Constant1/1 -> output1/1
  Constant2/1 -> output2/1
  Constant3/1 -> output3/1
  Constant5/1 -> output5/1
  Constant6/1 -> output6/1
  Constant7/1 -> output7/1
  Constant8/1 -> output8/1

== system FSAC2021/ROUTING/TO_DCAN/Subsystem/DIAG_VEH_INFO/Volt_Cmp_Mtr_Sts ==
  Volt_Cmp_Mtr_Sts : Inport
  Constant{1..4,6..8} (7 alike) : Constant  Value=0  OutDataTypeStr=uint8  SampleTime=-1
  Volt_Cmp_Mtr_StsRon : Rounding  Operator=round
  Volt_Cmp_Mtr_Sts_1sat : Saturate  UpperLimit=128  LowerLimit=0
  Volt_Cmp_Mtr_Sts_Convert : DataTypeConversion  OutDataTypeStr=uint8
  Volt_Cmp_Mtr_Sts_Convert1 : DataTypeConversion  OutDataTypeStr=uint32
  Volt_Cmp_Mtr_Sts_D : Product  Inputs=*/
  Volt_Cmp_Mtr_Sts_F : Constant  OutDataTypeStr=single
  Volt_Cmp_Mtr_Sts_L : simulink/Logic and Bit Operations/Bitwise Operator  logicop=AND  UseBitMask=on  BitMask=128  BitMaskRealWorld=Stored Integer
  Volt_Cmp_Mtr_Sts_O : Constant  Value=0  OutDataTypeStr=single
  Volt_Cmp_Mtr_Sts_S : ArithShift  BitShiftNumber=-7
  Volt_Cmp_Mtr_Sts_sat : Saturate  UpperLimit=1  LowerLimit=0
  Volt_Cmp_Mtr_Sts_st : Sum  Inputs=+-
  output1 : Outport
  output2 : Outport  Port=2
  output3 : Outport  Port=3
  output4 : Outport  Port=4
  output5 : Outport  Port=5
  output6 : Outport  Port=6
  output7 : Outport  Port=7
  output8 : Outport  Port=8
  wires:
  Volt_Cmp_Mtr_Sts/1 -> Volt_Cmp_Mtr_Sts_sat/1
  Volt_Cmp_Mtr_Sts_sat/1 -> Volt_Cmp_Mtr_Sts_st/1
  Volt_Cmp_Mtr_Sts_O/1 -> Volt_Cmp_Mtr_Sts_st/2
  Volt_Cmp_Mtr_Sts_st/1 -> Volt_Cmp_Mtr_Sts_D/1
  Volt_Cmp_Mtr_Sts_F/1 -> Volt_Cmp_Mtr_Sts_D/2
  Volt_Cmp_Mtr_Sts_D/1 -> Volt_Cmp_Mtr_StsRon/1
  Volt_Cmp_Mtr_StsRon/1 -> Volt_Cmp_Mtr_Sts_S/1
  Volt_Cmp_Mtr_Sts_S/1 -> Volt_Cmp_Mtr_Sts_1sat/1
  Volt_Cmp_Mtr_Sts_1sat/1 -> Volt_Cmp_Mtr_Sts_Convert1/1
  Volt_Cmp_Mtr_Sts_Convert1/1 -> Volt_Cmp_Mtr_Sts_L/1
  Volt_Cmp_Mtr_Sts_L/1 -> Volt_Cmp_Mtr_Sts_Convert/1
  Volt_Cmp_Mtr_Sts_Convert/1 -> output5/1
  Constant1/1 -> output1/1
  Constant2/1 -> output2/1
  Constant3/1 -> output3/1
  Constant4/1 -> output4/1
  Constant6/1 -> output6/1
  Constant7/1 -> output7/1
  Constant8/1 -> output8/1

== system FSAC2021/ROUTING/TO_DCAN/Subsystem/DIAG_VEH_SENSOR/BMS_Output_Volt ==
  BMS_Output_Volt : Inport
  BMS_Output_VoltRon : Rounding  Operator=round
  BMS_Output_Volt_1sat : Saturate  UpperLimit=255  LowerLimit=0
  BMS_Output_Volt_Convert : DataTypeConversion  OutDataTypeStr=uint8
  BMS_Output_Volt_Convert1 : DataTypeConversion  OutDataTypeStr=uint32
  BMS_Output_Volt_D : Product  Inputs=*/
  BMS_Output_Volt_F : Constant  OutDataTypeStr=single
  BMS_Output_Volt_L : simulink/Logic and Bit Operations/Bitwise Operator  logicop=AND  UseBitMask=on  BitMask=255  BitMaskRealWorld=Stored Integer
  BMS_Output_Volt_O : Constant  Value=0  OutDataTypeStr=single
  BMS_Output_Volt_S : ArithShift
  BMS_Output_Volt_sat : Saturate  UpperLimit=255  LowerLimit=0
  BMS_Output_Volt_st : Sum  Inputs=+-
  Constant{1..2,4..8} (7 alike) : Constant  Value=0  OutDataTypeStr=uint8  SampleTime=-1
  output1 : Outport
  output2 : Outport  Port=2
  output3 : Outport  Port=3
  output4 : Outport  Port=4
  output5 : Outport  Port=5
  output6 : Outport  Port=6
  output7 : Outport  Port=7
  output8 : Outport  Port=8
  wires:
  BMS_Output_Volt/1 -> BMS_Output_Volt_sat/1
  BMS_Output_Volt_sat/1 -> BMS_Output_Volt_st/1
  BMS_Output_Volt_O/1 -> BMS_Output_Volt_st/2
  BMS_Output_Volt_st/1 -> BMS_Output_Volt_D/1
  BMS_Output_Volt_F/1 -> BMS_Output_Volt_D/2
  BMS_Output_Volt_D/1 -> BMS_Output_VoltRon/1
  BMS_Output_VoltRon/1 -> BMS_Output_Volt_S/1
  BMS_Output_Volt_S/1 -> BMS_Output_Volt_1sat/1
  BMS_Output_Volt_1sat/1 -> BMS_Output_Volt_Convert1/1
  BMS_Output_Volt_Convert1/1 -> BMS_Output_Volt_L/1
  BMS_Output_Volt_L/1 -> BMS_Output_Volt_Convert/1
  BMS_Output_Volt_Convert/1 -> output3/1
  Constant1/1 -> output1/1
  Constant2/1 -> output2/1
  Constant4/1 -> output4/1
  Constant5/1 -> output5/1
  Constant6/1 -> output6/1
  Constant7/1 -> output7/1
  Constant8/1 -> output8/1

== system FSAC2021/ROUTING/TO_DCAN/Subsystem/DIAG_VEH_SENSOR/EBS_Gas_Prs_1 ==
  EBS_Gas_Prs_1 : Inport
  Constant{2..8} (7 alike) : Constant  Value=0  OutDataTypeStr=uint8  SampleTime=-1
  EBS_Gas_Prs_1Ron : Rounding  Operator=round
  EBS_Gas_Prs_1_1sat : Saturate  UpperLimit=15  LowerLimit=0
  EBS_Gas_Prs_1_Convert : DataTypeConversion  OutDataTypeStr=uint8
  EBS_Gas_Prs_1_Convert1 : DataTypeConversion  OutDataTypeStr=uint32
  EBS_Gas_Prs_1_D : Product  Inputs=*/
  EBS_Gas_Prs_1_F : Constant  Value=0.1  OutDataTypeStr=single
  EBS_Gas_Prs_1_L : simulink/Logic and Bit Operations/Bitwise Operator  logicop=AND  UseBitMask=on  BitMask=15  BitMaskRealWorld=Stored Integer
  EBS_Gas_Prs_1_O : Constant  Value=0  OutDataTypeStr=single
  EBS_Gas_Prs_1_S : ArithShift
  EBS_Gas_Prs_1_sat : Saturate  UpperLimit=1.5  LowerLimit=0
  EBS_Gas_Prs_1_st : Sum  Inputs=+-
  output1 : Outport
  output2 : Outport  Port=2
  output3 : Outport  Port=3
  output4 : Outport  Port=4
  output5 : Outport  Port=5
  output6 : Outport  Port=6
  output7 : Outport  Port=7
  output8 : Outport  Port=8
  wires:
  EBS_Gas_Prs_1/1 -> EBS_Gas_Prs_1_sat/1
  EBS_Gas_Prs_1_sat/1 -> EBS_Gas_Prs_1_st/1
  EBS_Gas_Prs_1_O/1 -> EBS_Gas_Prs_1_st/2
  EBS_Gas_Prs_1_st/1 -> EBS_Gas_Prs_1_D/1
  EBS_Gas_Prs_1_F/1 -> EBS_Gas_Prs_1_D/2
  EBS_Gas_Prs_1_D/1 -> EBS_Gas_Prs_1Ron/1
  EBS_Gas_Prs_1Ron/1 -> EBS_Gas_Prs_1_S/1
  EBS_Gas_Prs_1_S/1 -> EBS_Gas_Prs_1_1sat/1
  EBS_Gas_Prs_1_1sat/1 -> EBS_Gas_Prs_1_Convert1/1
  EBS_Gas_Prs_1_Convert1/1 -> EBS_Gas_Prs_1_L/1
  EBS_Gas_Prs_1_L/1 -> EBS_Gas_Prs_1_Convert/1
  EBS_Gas_Prs_1_Convert/1 -> output1/1
  Constant2/1 -> output2/1
  Constant3/1 -> output3/1
  Constant4/1 -> output4/1
  Constant5/1 -> output5/1
  Constant6/1 -> output6/1
  Constant7/1 -> output7/1
  Constant8/1 -> output8/1

== system FSAC2021/ROUTING/TO_DCAN/Subsystem/DIAG_VEH_SENSOR/EBS_Gas_Prs_2 ==
  EBS_Gas_Prs_2 : Inport
  Constant{2..8} (7 alike) : Constant  Value=0  OutDataTypeStr=uint8  SampleTime=-1
  EBS_Gas_Prs_2Ron : Rounding  Operator=round
  EBS_Gas_Prs_2_1sat : Saturate  UpperLimit=240  LowerLimit=0
  EBS_Gas_Prs_2_Convert : DataTypeConversion  OutDataTypeStr=uint8
  EBS_Gas_Prs_2_Convert1 : DataTypeConversion  OutDataTypeStr=uint32
  EBS_Gas_Prs_2_D : Product  Inputs=*/
  EBS_Gas_Prs_2_F : Constant  Value=0.1  OutDataTypeStr=single
  EBS_Gas_Prs_2_L : simulink/Logic and Bit Operations/Bitwise Operator  logicop=AND  UseBitMask=on  BitMask=240  BitMaskRealWorld=Stored Integer
  EBS_Gas_Prs_2_O : Constant  Value=0  OutDataTypeStr=single
  EBS_Gas_Prs_2_S : ArithShift  BitShiftNumber=-4
  EBS_Gas_Prs_2_sat : Saturate  UpperLimit=1.5  LowerLimit=0
  EBS_Gas_Prs_2_st : Sum  Inputs=+-
  output1 : Outport
  output2 : Outport  Port=2
  output3 : Outport  Port=3
  output4 : Outport  Port=4
  output5 : Outport  Port=5
  output6 : Outport  Port=6
  output7 : Outport  Port=7
  output8 : Outport  Port=8
  wires:
  EBS_Gas_Prs_2/1 -> EBS_Gas_Prs_2_sat/1
  EBS_Gas_Prs_2_sat/1 -> EBS_Gas_Prs_2_st/1
  EBS_Gas_Prs_2_O/1 -> EBS_Gas_Prs_2_st/2
  EBS_Gas_Prs_2_st/1 -> EBS_Gas_Prs_2_D/1
  EBS_Gas_Prs_2_F/1 -> EBS_Gas_Prs_2_D/2
  EBS_Gas_Prs_2_D/1 -> EBS_Gas_Prs_2Ron/1
  EBS_Gas_Prs_2Ron/1 -> EBS_Gas_Prs_2_S/1
  EBS_Gas_Prs_2_S/1 -> EBS_Gas_Prs_2_1sat/1
  EBS_Gas_Prs_2_1sat/1 -> EBS_Gas_Prs_2_Convert1/1
  EBS_Gas_Prs_2_Convert1/1 -> EBS_Gas_Prs_2_L/1
  EBS_Gas_Prs_2_L/1 -> EBS_Gas_Prs_2_Convert/1
  EBS_Gas_Prs_2_Convert/1 -> output1/1
  Constant2/1 -> output2/1
  Constant3/1 -> output3/1
  Constant4/1 -> output4/1
  Constant5/1 -> output5/1
  Constant6/1 -> output6/1
  Constant7/1 -> output7/1
  Constant8/1 -> output8/1
